simulink model "fortniteV2Sim"  (R2023b)
settings: Solver=FixedStepAuto  StartTime=0.0  StopTime=10.0  FixedStep=0.0001  RelTol=1e-3
values from neighbouring files (symbols this model uses):
  A = [0 1;-(kf)/(m) -(cf)/(m)]    [Lab6_damping.m]    (also in editer.m = zeros(1000,1); fortnite.m = [; fortniteV2.m = [; fortnite_DampPlot.m = [)
  B = randi([1,100])/100    [fitter.m]    (also in fortnite.m = [; fortniteV2.m = [; fortnite_DampPlot.m = [)
  C = randi([-15000,100])/10000    [fitter.m]    (also in fortniteV2.m = [1 0 0 0 0 0 0 0 0 0 0 0 0 0)
  D = randi([round(1000*(ymax-ymax*.2)),round(1000*(ymax+ymax*.2))])/1000    [fitter.m]    (also in fortniteV2.m = zeros(14,4))
undefined symbols (not defined in the file or in its folder): amp, freqq, pfl, pfr, prl, prr
settings Model: Creator=elija  LastModifiedBy=elija

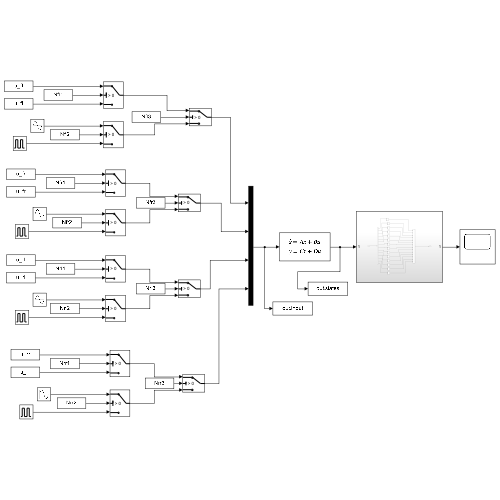
[thumbnail: Simulink's stored preview of the top-level diagram]
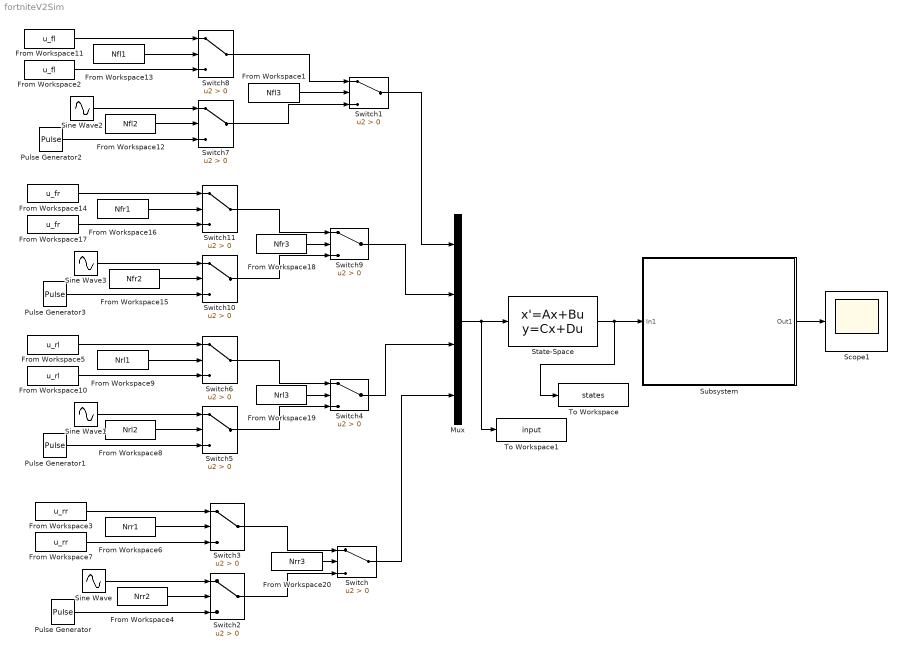
== system fortniteV2Sim ==
  From Workspace1 : FromWorkspace  VariableName=Nfl3
  From Workspace10 : FromWorkspace  VariableName=u_rl
  From Workspace11 : FromWorkspace  VariableName=u_fl
  From Workspace12 : FromWorkspace  VariableName=Nfl2
  From Workspace13 : FromWorkspace  VariableName=Nfl1
  From Workspace14 : FromWorkspace  VariableName=u_fr
  From Workspace15 : FromWorkspace  VariableName=Nfr2
  From Workspace16 : FromWorkspace  VariableName=Nfr1
  From Workspace17 : FromWorkspace  VariableName=u_fr
  From Workspace18 : FromWorkspace  VariableName=Nfr3
  From Workspace19 : FromWorkspace  VariableName=Nrl3
  From Workspace2 : FromWorkspace  VariableName=u_fl
  From Workspace20 : FromWorkspace  VariableName=Nrr3
  From Workspace3 : FromWorkspace  VariableName=u_rr
  From Workspace4 : FromWorkspace  VariableName=Nrr2
  From Workspace5 : FromWorkspace  VariableName=u_rl
  From Workspace6 : FromWorkspace  VariableName=Nrr1
  From Workspace7 : FromWorkspace  VariableName=u_rr
  From Workspace8 : FromWorkspace  VariableName=Nrl2
  From Workspace9 : FromWorkspace  VariableName=Nrl1
  Mux : Mux
  Pulse Generator : DiscretePulseGenerator  PulseType=Time based  Amplitude=amp  Period=freqq  PulseWidth=5  PhaseDelay=prr
  Pulse Generator1 : DiscretePulseGenerator  PulseType=Time based  Amplitude=amp  Period=freqq  PulseWidth=5  PhaseDelay=prl
  Pulse Generator2 : DiscretePulseGenerator  PulseType=Time based  Amplitude=amp  Period=freqq  PulseWidth=5  PhaseDelay=pfl
  Pulse Generator3 : DiscretePulseGenerator  PulseType=Time based  Amplitude=amp  Period=freqq  PulseWidth=5  PhaseDelay=pfr
  Scope1 : Scope
  Sine Wave : Sin  Amplitude=amp  Frequency=freqq  Phase=prr  SampleTime=0
  Sine Wave1 : Sin  Amplitude=amp  Frequency=freqq  Phase=prl  SampleTime=0
  Sine Wave2 : Sin  Amplitude=amp  Frequency=freqq  Phase=pfl  SampleTime=0
  Sine Wave3 : Sin  Amplitude=amp  Frequency=freqq  Phase=pfr  SampleTime=0
  State-Space : StateSpace  A=A  B=B  C=C  D=D  InitialCondition=0
  Subsystem : Subsystem
  Switch{,1..11} (12 alike) : Switch  Criteria=u2 > Threshold  OutDataTypeStr=Inherit: Inherit via back propagation  SaturateOnIntegerOverflow=off  InputSameDT=off
  To Workspace : ToWorkspace  VariableName=states  SaveFormat=Timeseries  SampleTime=-1
  To Workspace1 : ToWorkspace  VariableName=input  SaveFormat=Timeseries  SampleTime=-1
  wires:
  From Workspace3/1 -> Switch3/1
  Mux/1 -> To Workspace1/1, State-Space/1
  State-Space/1 -> To Workspace/1, Subsystem/1(In1)
  Subsystem/1(Out1) -> Scope1/1
  Switch/1 -> Mux/4
  Switch2/1 -> Switch/3
  Sine Wave/1 -> Switch2/1
  Pulse Generator/1 -> Switch2/3
  From Workspace4/1 -> Switch2/2
  Switch3/1 -> Switch/1
  From Workspace6/1 -> Switch3/2
  From Workspace7/1 -> Switch3/3
  Switch6/1 -> Switch4/1
  From Workspace5/1 -> Switch6/1
  From Workspace9/1 -> Switch6/2
  Sine Wave1/1 -> Switch5/1
  Switch5/1 -> Switch4/3
  From Workspace10/1 -> Switch6/3
  From Workspace8/1 -> Switch5/2
  Switch4/1 -> Mux/3
  Pulse Generator1/1 -> Switch5/3
  From Workspace12/1 -> Switch7/2
  Sine Wave2/1 -> Switch7/1
  Pulse Generator2/1 -> Switch7/3
  From Workspace2/1 -> Switch8/3
  From Workspace13/1 -> Switch8/2
  Switch7/1 -> Switch1/3
  From Workspace11/1 -> Switch8/1
  Switch8/1 -> Switch1/1
  Switch1/1 -> Mux/1
  From Workspace14/1 -> Switch11/1
  Switch11/1 -> Switch9/1
  Switch10/1 -> Switch9/3
  Pulse Generator3/1 -> Switch10/3
  Switch9/1 -> Mux/2
  From Workspace15/1 -> Switch10/2
  Sine Wave3/1 -> Switch10/1
  From Workspace16/1 -> Switch11/2
  From Workspace17/1 -> Switch11/3
  From Workspace1/1 -> Switch1/2
  From Workspace18/1 -> Switch9/2
  From Workspace19/1 -> Switch4/2
  From Workspace20/1 -> Switch/2

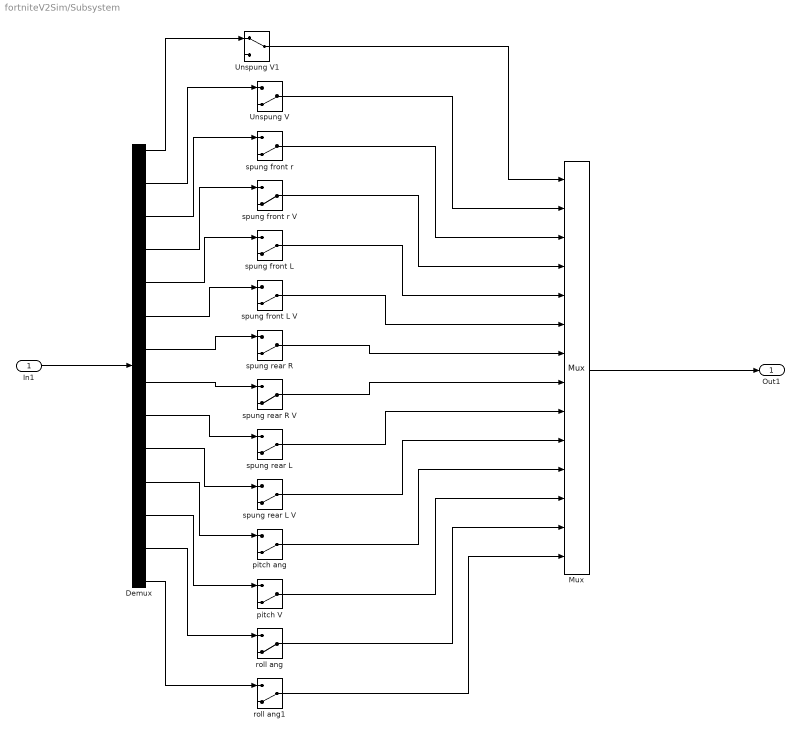
== system fortniteV2Sim/Subsystem ==
  In1 : Inport
  Demux : Demux  Outputs=14
  Mux : Mux  Inputs=14
  Unspung V : ManualSwitch  CurrentSetting=0
  Unspung V1 : ManualSwitch
  pitch V : ManualSwitch  CurrentSetting=0
  pitch ang : ManualSwitch  CurrentSetting=0
  roll ang : ManualSwitch  CurrentSetting=0
  roll ang1 : ManualSwitch  CurrentSetting=0
  spung front L : ManualSwitch  CurrentSetting=0
  spung front L V : ManualSwitch  CurrentSetting=0
  spung front r : ManualSwitch  CurrentSetting=0
  spung front r V : ManualSwitch  CurrentSetting=0
  spung rear L : ManualSwitch  CurrentSetting=0
  spung rear L V : ManualSwitch  CurrentSetting=0
  spung rear R : ManualSwitch  CurrentSetting=0
  spung rear R V : ManualSwitch  CurrentSetting=0
  Out1 : Outport
  wires:
  In1/1 -> Demux/1
  spung rear L/1 -> Mux/9
  spung rear R/1 -> Mux/7
  pitch ang/1 -> Mux/11
  Demux/12 -> pitch V/1
  Demux/6 -> spung front L V/1
  Demux/5 -> spung front L/1
  Demux/10 -> spung rear L V/1
  Demux/2 -> Unspung V/1
  Demux/9 -> spung rear L/1
  roll ang/1 -> Mux/13
  Demux/3 -> spung front r/1
  spung front L V/1 -> Mux/6
  spung front L/1 -> Mux/5
  Demux/4 -> spung front r V/1
  Demux/13 -> roll ang/1
  roll ang1/1 -> Mux/14
  Unspung V/1 -> Mux/2
  Demux/8 -> spung rear R V/1
  Demux/7 -> spung rear R/1
  Unspung V1/1 -> Mux/1
  pitch V/1 -> Mux/12
  spung front r/1 -> Mux/3
  spung rear L V/1 -> Mux/10
  spung front r V/1 -> Mux/4
  spung rear R V/1 -> Mux/8
  Demux/11 -> pitch ang/1
  Demux/1 -> Unspung V1/1
  Mux/1 -> Out1/1
  Demux/14 -> roll ang1/1
